simulink model "SerialCommIn_V1"  (R2017b)
settings: Solver=FixedStepAuto  StartTime=0.0  StopTime=inf  FixedStep=0.001  RelTol=1e-3  EnableMultiTasking=on
undefined symbols (not defined in the file): D10, D11, D12, D2, D5, D8, D9, PTA0, PTA2, PTB9, PTC4, PTD0, PTD2, PTD3
libraries: frdmk64flib x11
settings Model: ExtModeTrigDuration=5  Creator=montema2  LastModifiedBy=brydoa1
settings OptimizationCC: PassReuseOutputArgsAs=Individual arguments  MaxStackSize=64
settings DebuggingCC: ParameterTunabilityLossMsg=error
settings HardwareCC: ProdBitPerPointer=32  ProdBitPerSizeT=32  ProdBitPerPtrDiffT=32  ProdLargestAtomicInteger=Long  ProdLargestAtomicFloat=Double  ProdWordSize=32  ProdHWDeviceType=ARM Compatible->ARM Cortex
settings SFSimCC: MATLABDynamicMemAlloc=off
settings RTWCC: SystemTargetFile=ert.tlc  HardwareBoard=NXP FRDM-K64F  TemplateMakefile=ert_default_tmf  GenerateReport=on  Toolchain=GNU Tools for ARM Embedded Processors  IncludeHyperlinkInReport=on  LaunchReport=on  GenerateTraceInfo=on  GenerateTraceReport=on  GenerateTraceReportSl=on  GenerateTraceReportSf=on  GenerateTraceReportEml=on
settings CodeAppCC: ForceParamTrailComments=on  IgnoreCustomStorageClasses=off  OperatorAnnotations=on  SimulinkDataObjDesc=on  SFDataObjDesc=on  InsertBlockDesc=on

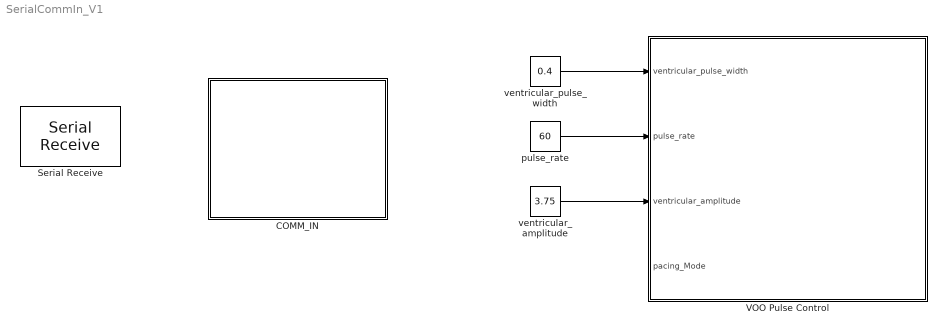
== system SerialCommIn_V1 ==
  COMM_IN : Stateflow chart  TreatAsAtomicUnit=on
  Serial Receive : frdmk64flib/Serial Receive  SCIModule=0  Baudrate=uint32(9600)  Parity=None  StopBits=1  HardwareFlowControl=None  ByteOrder=LittleEndian  DataType=uint8  DataLength=10  BlockingMode=off  OutputStatus=on  SampleTime=-1
      settings: SourceProductName=Simulink Coder Support Package for NXP FRDM-K64F Board
  VOO Pulse Control : Subsystem
  pulse_rate : Constant  Value=60  OutMin=[50]  OutMax=[175]
  ventricular_amplitude : Constant  Value=3.75
  ventricular_pulse_width : Constant  Value=0.4
  wires:
  ventricular_pulse_width/1 -> VOO Pulse Control/1(ventricular_pulse_width)
  pulse_rate/1 -> VOO Pulse Control/2(pulse_rate)
  ventricular_amplitude/1 -> VOO Pulse Control/3(ventricular_amplitude)

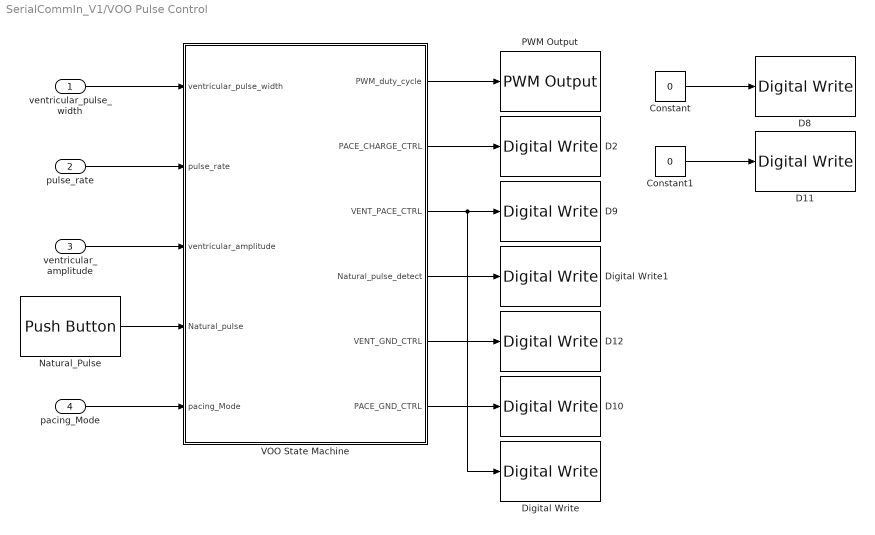
== system SerialCommIn_V1/VOO Pulse Control ==
  ventricular_pulse_width : Inport
  pulse_rate : Inport  Port=2
  ventricular_amplitude : Inport  Port=3
  pacing_Mode : Inport  Port=4
  Constant : Constant  Value=0
  Constant1 : Constant  Value=0
  D10 : frdmk64flib/Digital Write  Whichpin=PTD0 (D10)
      settings: SourceProductName=Simulink Coder Support Package for NXP FRDM-K64F Board
  D11 : frdmk64flib/Digital Write  Whichpin=PTD2 (D11)
      settings: SourceProductName=Simulink Coder Support Package for NXP FRDM-K64F Board
  D12 : frdmk64flib/Digital Write  Whichpin=PTD3 (D12)
      settings: SourceProductName=Simulink Coder Support Package for NXP FRDM-K64F Board
  D2 : frdmk64flib/Digital Write  Whichpin=PTB9 (D2)
      settings: SourceProductName=Simulink Coder Support Package for NXP FRDM-K64F Board
  D8 : frdmk64flib/Digital Write  Whichpin=PTA0 (D8)
      settings: SourceProductName=Simulink Coder Support Package for NXP FRDM-K64F Board
  D9 : frdmk64flib/Digital Write  Whichpin=PTC4 (D9)
      settings: SourceProductName=Simulink Coder Support Package for NXP FRDM-K64F Board
  Digital Write : frdmk64flib/Digital Write  Whichpin=RED_LED
      settings: SourceProductName=Simulink Coder Support Package for NXP FRDM-K64F Board
  Digital Write1 : frdmk64flib/Digital Write  Whichpin=BLUE_LED
      settings: SourceProductName=Simulink Coder Support Package for NXP FRDM-K64F Board
  Natural_Pulse : frdmk64flib/Push Button  Whichswitch=SW2  SampleTime1=-1
      settings: SourceProductName=Simulink Coder Support Package for NXP FRDM-K64F Board
  PWM Output : frdmk64flib/PWM Output  Whichpin=PTA2 (D5)  InitialFrequency=1000  InitialDutyCycle=0
      settings: SourceProductName=Simulink Coder Support Package for NXP FRDM-K64F Board
  VOO State Machine : Stateflow chart  TreatAsAtomicUnit=on
  wires:
  ventricular_pulse_width/1 -> VOO State Machine/1(ventricular_pulse_width)
  VOO State Machine/1(PWM_duty_cycle) -> PWM Output/1
  VOO State Machine/3(VENT_PACE_CTRL) -> Digital Write/1, D9/1
  pulse_rate/1 -> VOO State Machine/2(pulse_rate)
  VOO State Machine/2(PACE_CHARGE_CTRL) -> D2/1
  VOO State Machine/5(VENT_GND_CTRL) -> D12/1
  VOO State Machine/6(PACE_GND_CTRL) -> D10/1
  Constant/1 -> D8/1
  Constant1/1 -> D11/1
  Natural_Pulse/1 -> VOO State Machine/4(Natural_pulse)
  VOO State Machine/4(Natural_pulse_detect) -> Digital Write1/1
  ventricular_amplitude/1 -> VOO State Machine/3(ventricular_amplitude)
  pacing_Mode/1 -> VOO State Machine/5(pacing_Mode)

== stateflow chart SerialCommIn_V1/COMM_IN ==
  state INITIAL
    %Set intial values of parameters
    %VOO mode?
    entry: rateAdapt = 0;
    vent_Pulse_Width = 10; %milliseconds
    atr_Pulse_Width = 10;
    min_Rate_Lim = 60; %bpm
    vent_Pulse_Amp = 3.5; %volts
    atr_Pulse_Amp = 3.5;
  state VENT_CURRENT_IN
    entry:
    PACE_CHARGE_CTRL=false;
    VENT_GND_CTRL=false;
    VENT_PACE_CTRL=true;
  state STANDBY
    %Wait for signal from DCM
  state VENTRICLE_INIT
    entry:VENT_PACE_CTRL=false;
    VENT_GND_CTRL=true;
    ATR_PACE_CTRL=false;
    ATR_GND_CTRL=true;
    PACE_CHARGE_CTRL=true;
    PACE_GND_CTRL=true;
  note: double check ATR_GND_CTRL state
  state VENT_PULSE_SENSE
  note: double check VENT_GND_CTRL state
  state ATRIAL_INIT
    entry:VENT_PACE_CTRL=false;
    VENT_GND_CTRL=true;
    ATR_PACE_CTRL=false;
    ATR_GND_CTRL=true;
    PACE_CHARGE_CTRL=true;
    PACE_GND_CTRL=true;
  state PARAM_INIT
    entry: pace_Mode = rxdata(0);
    min_Rate_Lim = rxdata(1);
    max_Rate_Lim = rxdata(2);
    max_Sensor_Rate = rxdata(3);
    fix_AV_Delay = rxdata(4);
    dyn_AV_Delay = rxdata(5);
    min_Dyn_AV_Delay = rxdata(6);
    sensed_AV_Delay_Offset_State = rxdata(7);
    sensed_AV_Delay_Offset_Val = rxdata(8);
    vent_Pulse_Amp = ((rxdata(9)/5)*100);
    atr_Pulse_Amp = ((rxdata(10)/5)*100);
    vent_Pulse_Width = rxdata(11);
    atr_Pulse_Width = rxdata(12);
    vent_Sens = rxdata(13);
    atr_Sens = rxdata(14);
    vent_Ref_Per = rxdata(15);
    atr_Ref_Per = rxdata(16);
    PVARP = rxdata(17);
    PVARP_Ext_State = rxdata(18);
    PVARP_Ext_Val = rxdata(19);
    hyst_State = rxdata(20);
    hyst_Rate_Lim = rxdata(21);
    rate_Smooth_State = rxdata(22);
    rate_Smooth_Val = rxdata(23);
    ATR_State = rxdata(24);
    ATR_Duration = rxdata(25);
    ATR_Fallback = rxdata(26);
    activity_Thresh = rxdata(27);
    reaction_Time = rxdata(28);
    response_Factor = rxdata(29);
    recovery_Time = rxdata(30);
  state VENT_CURRENT_OUT
    entry:
    VENT_PACE_CTRL=false;
    PACE_CHARGE_CTRL=true;
    VENT_GND_CTRL=true;
  state VVI_INIT [commented out]
    entry:VENT_PACE_CTRL=false;
    VENT_GND_CTRL=true;
    PACE_CHARGE_CTRL=true;
    PACE_GND_CTRL=true;
  state AAI_INIT [commented out]
    entry:ATR_PACE_CTRL=false;
    ATR_GND_CTRL=true;
    PACE_CHARGE_CTRL=true;
    PACE_GND_CTRL=true;
  state ATR_CURRENT_IN
    entry:
    PACE_CHARGE_CTRL=false;
    ATR_GND_CTRL=false;
    ATR_PACE_CTRL=true;
  state DUAL_INIT
    entry:VENT_PACE_CTRL=false;
    VENT_GND_CTRL=true;
    ATR_PACE_CTRL=false;
    ATR_GND_CTRL=true;
    PACE_CHARGE_CTRL=true;
    PACE_GND_CTRL=true;
  state ATR_PULSE_SENSE
  state DDD_INIT
  state ATR_CURRENT_OUT
    entry:
    ATR_PACE_CTRL=false;
    PACE_CHARGE_CTRL=true;
    ATR_GND_CTRL=true;
  (default) -> INITIAL
  ATR_CURRENT_OUT -> VENT_CURRENT_IN [order 2] : [(pace_Mode ==  5 || pace_Mode ==11)&&(after((fix_AV_Delay),msec))]
  VENTRICLE_INIT -> VENT_CURRENT_IN : [after(((min_Rate_Lim)*1000),msec)]
  VENT_CURRENT_IN -> VENT_PULSE_SENSE [order 2] : [(natural_Pace == 1)&&(pace_Mode == 3|| pace_Mode == 4 || pace_Mode == 6 || pace_Mode == 9 || pace_Mode == 10 || pace_Mode == 12)]
  INITIAL -> STANDBY
  VENT_CURRENT_OUT -> VENT_CURRENT_IN [order 1] : [(pace_Mode == 1 || pace_Mode ==3 || pace_Mode == 7 || pace_Mode == 9)&&(after(((60/min_Rate_Lim)*1000)-(vent_Pulse_Width),msec))]
  VENT_CURRENT_IN -> VENT_CURRENT_OUT [order 1] : [after((vent_Pulse_Width),msec)]
  (junction 5) -> STANDBY [order 2]
  STANDBY -> (junction 5) : [status == 0]
  (junction 7) -> VENTRICLE_INIT [order 1] : [pace_Mode ==1 || pace_Mode == 3 || pace_Mode ==7 || pace_Mode == 9]
  (junction 5) -> (junction 38) [order 1] : [rxdata(0) > 0 && rxdata(1) < 13 ]
  (junction 38) -> PARAM_INIT : [rxdata(0) > 6]{rateAdapt = 1}
  VENT_CURRENT_OUT -> VENT_PULSE_SENSE [order 3]
  ATRIAL_INIT -> ATR_CURRENT_IN : [after(((min_Rate_Lim)*1000),msec)]
  (junction 7) -> ATRIAL_INIT [order 2] : [pace_Mode ==2 || pace_Mode == 4 || pace_Mode ==8 || pace_Mode ==10]
  (junction 7) -> VVI_INIT [commented out] : [pace_Mode ==3 || pace_Mode == 9]
  VENT_CURRENT_OUT -> ATR_CURRENT_IN [order 2] : [(pace_Mode ==  5 || pace_Mode ==11)&&(after(((60/min_Rate_Lim)*1000)-(vent_Pulse_Width)-(atr_Pulse_width)-(fix_AV_Delay),msec))]
  PARAM_INIT -> (junction 7)
  (junction 7) -> AAI_INIT [commented out] : [pace_Mode ==4 || pace_Mode ==10 ]
  (junction 7) -> DUAL_INIT [order 3] : [pace_Mode ==5 || pace_Mode == 11]
  (junction 7) -> DDD_INIT [order 4] : [pace_Mode ==6 || pace_Mode ==12 ]
  DUAL_INIT -> ATR_CURRENT_IN : [after(((min_Rate_Lim)*1000),msec)]
  DDD_INIT -> ATR_CURRENT_IN : [after(((min_Rate_Lim)*1000),msec)]
  ATR_CURRENT_OUT -> ATR_CURRENT_IN [order 1] : [(pace_Mode == 2 || pace_Mode == 4 || pace_Mode == 8 || pace_Mode == 10)&&(after(((60/min_Rate_Lim)*1000)-(atr_Pulse_Width),msec)) ]
  ATR_CURRENT_IN -> ATR_CURRENT_OUT : [after((atr_Pulse_Width),msec)]

== stateflow chart SerialCommIn_V1/VOO Pulse Control/VOO State Machine ==
  note: Switch States:
      | true=closed
      | false=open
  state current_into_heart
    entry:
    PACE_CHARGE_CTRL=false;
    VENT_GND_CTRL=false;
    VENT_PACE_CTRL=true;
  state start_state
    entry:VENT_PACE_CTRL=false;
    VENT_GND_CTRL=true;
    PACE_CHARGE_CTRL=true;
    PACE_GND_CTRL=true;
    PWM_duty_cycle=((ventricular_amplitude/5)*100);
  state current_out_of_heart
    entry:
    VENT_PACE_CTRL=false;
    PACE_CHARGE_CTRL=true;
    VENT_GND_CTRL=true;
  state natural_pace
    entry: Natural_pulse_detect=true;
    exit: Natural_pulse_detect=false;
  (default) -> start_state
  start_state -> current_into_heart [order 1] : [after(((60/pulse_rate)*1000),msec)]
  current_into_heart -> natural_pace [order 2] : [Natural_pulse==true]
  start_state -> natural_pace [order 2] : [Natural_pulse==true]
  natural_pace -> start_state : [Natural_pulse==false]
  current_into_heart -> current_out_of_heart [order 1] : [after((ventricular_pulse_width),msec)]
  current_out_of_heart -> current_into_heart [order 1] : [after(((60/pulse_rate)*1000)-(ventricular_pulse_width),msec)]
  current_out_of_heart -> natural_pace [order 2] : [Natural_pulse==true]
  data: ventricular_pulse_width input double; pulse_rate input double; ventricular_amplitude input double; PWM_duty_cycle output double [0..100]; PACE_CHARGE_CTRL output boolean; VENT_PACE_CTRL output boolean; Natural_pulse_detect output; VENT_GND_CTRL output boolean; PACE_GND_CTRL output boolean; Natural_pulse input boolean; pacing_Mode input uint8
